simulink model "controlTypes"  (R2021a)
settings: Solver=VariableStepAuto  StartTime=0.0  StopTime=10  RelTol=1e-3
libraries: mcbcontrolslib x3, simulink x1
settings Model: Creator=Maxim  LastModifiedBy=Max

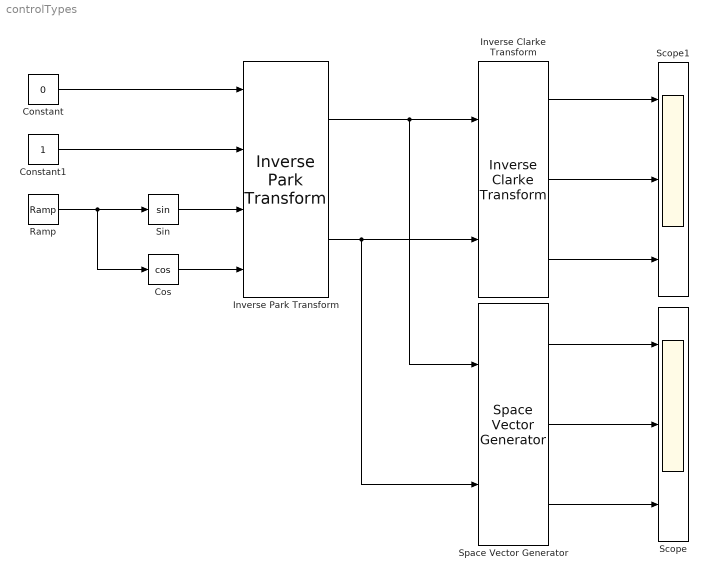
== system controlTypes ==
  Constant : Constant  Value=0
  Constant1 : Constant
  Cos : Trigonometry  Operator=cos
  Inverse Clarke Transform : mcbcontrolslib/Inverse Clarke Transform
      settings: SourceProductBaseCode=MT
  Inverse Park Transform : mcbcontrolslib/Inverse Park Transform  AxisAlignment=D-axis
  Ramp : simulink/Sources/Ramp  slope=pi*60/180  start=0  InitialOutput=0
  Scope : Scope  NumInputPorts=3
  Scope1 : Scope  NumInputPorts=3
  Sin : Trigonometry
  Space Vector Generator : mcbcontrolslib/Space Vector Generator
      settings: SourceProductBaseCode=MT
  wires:
  Inverse Park Transform/2 -> Space Vector Generator/2, Inverse Clarke Transform/2
  Inverse Park Transform/1 -> Space Vector Generator/1, Inverse Clarke Transform/1
  Constant1/1 -> Inverse Park Transform/2
  Sin/1 -> Inverse Park Transform/3
  Cos/1 -> Inverse Park Transform/4
  Ramp/1 -> Cos/1, Sin/1
  Space Vector Generator/1 -> Scope/1
  Space Vector Generator/2 -> Scope/2
  Space Vector Generator/3 -> Scope/3
  Inverse Clarke Transform/1 -> Scope1/1
  Inverse Clarke Transform/2 -> Scope1/2
  Inverse Clarke Transform/3 -> Scope1/3
  Constant/1 -> Inverse Park Transform/1
